simulink model "project"  (R2021b)
settings: Solver=VariableStepAuto  StartTime=0.0  StopTime=10.0  RelTol=1e-3
settings Model: DataDictionary=DesignData.sldd  Creator=barbora.fedova  LastModifiedBy=barbora.fedova

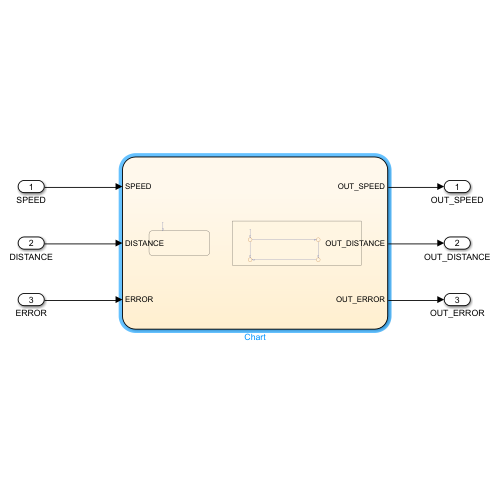
[thumbnail: Simulink's stored preview of the top-level diagram]
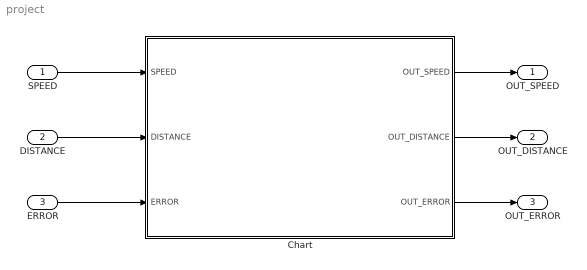
== system project ==
  SPEED : Inport
  DISTANCE : Inport  Port=2
  ERROR : Inport  Port=3  OutDataTypeStr=Enum: ERROR_E
  Chart : Stateflow chart  TreatAsAtomicUnit=on
      settings: PortSchema="{\"entries\":[{\"content\":{\"sides\":[{\"content\":{\"connectorIds\":[\"In3\",\"In1\",\"In2\"]},\"type\":\"ConnectorPlacement.EquallySpacedRectSide\",\"uuid\":\"42b3525d-4490-4846-b2f1-c9d6093cf098\"},{\"content\":{\"connectorIds\":[\"Out1\",\"Out2\",\"Out3\"],\"side\":\"RIGHT\"},\"type\":\"ConnectorPlacement.EquallySpacedRectSide\",\"uuid\":\"2d567bfa-d0a1-4dd3-8165-1e9840356359\"},{\"content\":{\"connectorIds\":[],\"side\":\"TOP\"},\"type\":\"ConnectorPlacement.EquallySpacedRectSide\",\"uuid\":\"55097e24-5744-4b46-841e-7cd92f33f85f\"}]},\"type\":\"ConnectorPlacement.EquallySpacedConnector\",\"uuid\":\"858bfe1c-7203-4d29-ab79-517451ce654d\"}],\"packageUris\":[\"http://schema.mathworks.com/mf0/Connector/R2020b\"],\"version\":\"1.0\"}"
  OUT_SPEED : Outport
  OUT_DISTANCE : Outport  Port=2
  OUT_ERROR : Outport  Port=3
  wires:
  Chart/2(OUT_DISTANCE) -> OUT_DISTANCE/1
  Chart/1(OUT_SPEED) -> OUT_SPEED/1
  Chart/3(OUT_ERROR) -> OUT_ERROR/1
  DISTANCE/1 -> Chart/1(DISTANCE)
  ERROR/1 -> Chart/2(ERROR)
  SPEED/1 -> Chart/3(SPEED)

== stateflow chart project/Chart ==
  state ret_OUT_SPEED = calculateSpeed [function]
    (default) -> (junction 14)
    (junction 14) -> (junction 19) [order 2]
    (junction 14) -> (junction 17) [order 1] : [SPEED >= SPEED_THRESHOLD]
        | {ret_OUT_SPEED = 5;}
    (junction 19) -> (junction 20) : {ret_OUT_SPEED = 0;}
    (junction 20) -> (junction 17)
  state STATE_INIT
    du:
    OUT_SPEED = calculateSpeed();
    OUT_DISTANCE = DISTANCE;
    OUT_ERROR = ERROR;
  (default) -> STATE_INIT
  data: ret_OUT_SPEED function_output; OUT_SPEED output; OUT_DISTANCE output; OUT_ERROR output; DISTANCE input; ERROR input; SPEED input; SPEED_THRESHOLD parameter
